simulink model "sf_if"  (R2017b)
settings: Solver=ode45  StartTime=0.0  StopTime=10.0  MaxStep=.05  RelTol=1e-3  EnableMultiTasking=on
libraries: simulink x1
settings Model: FPTRunName=Active  ExtModeAutoUpdateStatusClock=off  Creator=The MathWorks, Inc.  LastModifiedBy=The MathWorks, Inc.
settings DataIOCC: LimitDataPoints=on  SaveFormat=Array  SignalLoggingName=sigsOut
settings OptimizationCC: ExpressionDepthLimit=2147483647  InitFltsAndDblsToZero=on  EfficientMapNaN2IntZero=off  LifeSpan=inf
settings DebuggingCC: SaveWithParameterizedLinksMsg=none  UnderspecifiedInitializationDetection=Classic  MergeDetectMultiDrivingBlocksExec=none  SignalResolutionControl=TryResolveAllWithWarning  MultiTaskDSMMsg=warning  MultiTaskCondExecSysMsg=none  FcnCallInpInsideContextMsg=warning  StateNameClashWarn=warning  StrictBusMsg=None  SFUnexpectedBacktrackingDiag=warning  SFNoUnconditionalDefaultTransitionDiag=warning  SFExecutionAtInitializationDiag=none
settings HardwareCC: ProdBitPerPointer=32  ProdBitPerSizeT=32  ProdBitPerPtrDiffT=32  ProdLargestAtomicFloat=None  ProdIntDivRoundTo=Undefined  ProdEndianess=Unspecified  ProdWordSize=32  ProdHWDeviceType=32-bit Generic  TargetUnknown=on
settings ModelReferenceCC: PropagateSignalLabelsOutOfModel=off
settings SFSimCC: SimParseCustomCode=off
settings CodeAppCC: StateflowObjectComments=on
settings GRTTargetCC: TargetFcnLib=ansi_tfl_tmw.mat  TargetLangStandard=C89/C90 (ANSI)  GeneratePreprocessorConditionals=Disable all  CombineOutputUpdateFcns=off  GRTInterface=on
settings ConfigComp: CovMetricSettings=dcmtr  CovHtmlReporting=on  CovSaveCumulativeToWorkspaceVar=on  CovSaveSingleToWorkspaceVar=on  CovExternalEMLEnable=off  CovSFcnEnable=off

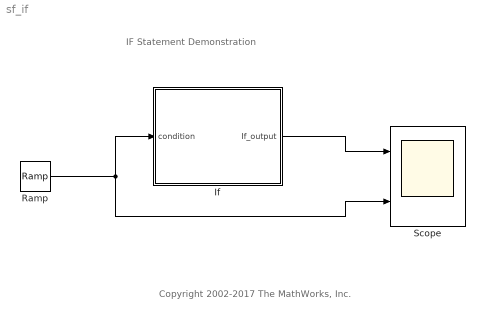
== system sf_if ==
  note: IF Statement Demonstration
  note: Copyright 2002-2017 The MathWorks, Inc.
  If : Stateflow chart  TreatAsAtomicUnit=on
  Ramp : simulink/Sources/Ramp  slope=10  start=0  X0=0
  Scope : Scope  NumInputPorts=2
  wires:
  Ramp/1 -> If/1(condition), Scope/2
  If/1(If_output) -> Scope/1

== stateflow chart sf_if/If ==
  note: Equivalent M-Code:
      |
      | if condition <= 20
      |     If_output = condition^2;
      | elseif condition > 20 & condition <=70
      |    If_output = 50*sin(condition)
      | else
      |    If_output = condition;
      | end
  (default) -> (junction 12)
  (junction 12) -> (junction 15) [order 1] : [condition<=20]
  (junction 12) -> (junction 14) [order 2]
  (junction 15) -> (junction 16) : {If_output=power(condition,2);}
  (junction 14) -> (junction 17) [order 1] : [condition>20 && condition<=70]
  (junction 14) -> (junction 13) [order 2] : {If_output=condition;}
  (junction 17) -> (junction 18) : {If_output=50*sin(condition);}
  (junction 18) -> (junction 13)
  (junction 16) -> (junction 18)
  (junction 13) -> (junction 19)
  data: condition input double; If_output output double
